simulink model "MPC"  (R2018a)
settings: Solver=VariableStepAuto  StartTime=0.0  StopTime=30  RelTol=1e-3
values from neighbouring files (symbols this model uses):
  I = 2500    [params.m]
  Kf = 55000    [params.m]
  Kr = 60000    [params.m]
  lf = 1.1    [params.m]
  lr = 1.6    [params.m]
  m = 1500    [params.m]
  n = 18.7    [params.m]
libraries: mpclib x1
settings Model: Creator=aoki-soya  LastModifiedBy=aoki-soya

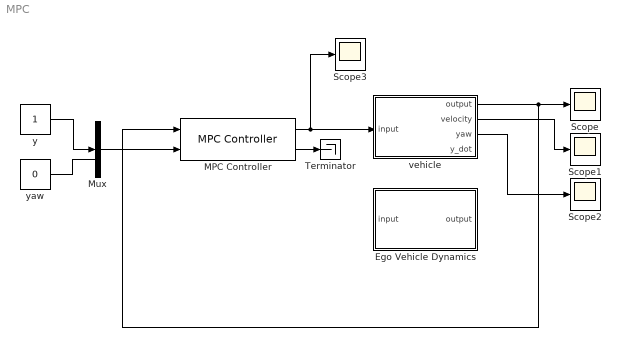
== system MPC ==
  Ego Vehicle Dynamics : Subsystem
  MPC Controller : mpclib/MPC Controller  SCDEnableBlockLinearizationSpecification=on  mpcobj=mpc1  is_multiple=0  enable_value=0  return_u0=off  updateMPCinCallerWorkspace=on  ref_from_ws=off  ref_signal_name=[]  ref_preview=off  md_from_ws=off  md_signal_name=[]  md_preview=off  from_project=off  project_file=MPCtask.mat  md_inport=off  mv_inport=off  cost_outport=on  return_sequence=off  return_qpstatus=off  return_state=off  state_inport=off  lims_inport=off  cc_inport=off  ywt_inport=off  is_designfromscratch=0  uwt_inport=off  duwt_inport=off  rhoeps_inport=off  uref_inport=off  n_ts=0.1  n_p=10  n_mv=2  n_md=0  n_ud=0  n_mo=1  n_uo=0  BlockDataType=double  SampleTimeInherited=off  switch_inport=off
  Mux : Mux  Inputs=1
  Scope{,1..3} (4 alike) : Scope
  Terminator : Terminator
  vehicle : Subsystem
  y : Constant
  yaw : Constant  Value=0
  wires:
  MPC Controller/1 -> Scope3/1, vehicle/1(input)
  vehicle/1(output) -> MPC Controller/1, Scope/1
  Mux/1 -> MPC Controller/2
  y/1 -> Mux/1
  yaw/1 -> ?
  MPC Controller/2 -> Terminator/1
  vehicle/2(velocity) -> Scope1/1
  vehicle/3(yaw) -> Scope2/1

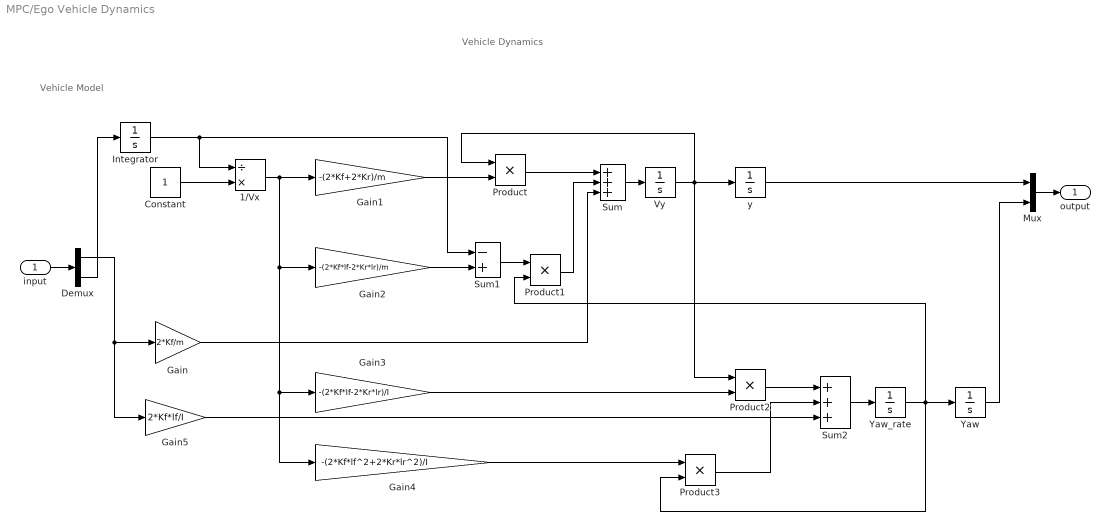
== system MPC/Ego Vehicle Dynamics ==
  note: Vehicle Model
  note: Vehicle Dynamics
  input : Inport
  1/Vx : Product  Inputs=/*
  Constant : Constant
  Demux : Demux  Outputs=2
  Gain : Gain  Gain=2*Kf/m
  Gain1 : Gain  Gain=-(2*Kf+2*Kr)/m
  Gain2 : Gain  Gain=-(2*Kf*lf-2*Kr*lr)/m
  Gain3 : Gain  Gain=-(2*Kf*lf-2*Kr*lr)/I
  Gain4 : Gain  Gain=-(2*Kf*lf^2+2*Kr*lr^2)/I
  Gain5 : Gain  Gain=2*Kf*lf/I
  Integrator : Integrator  InitialCondition=0.1  LimitOutput=on  LowerSaturationLimit=0.01
  Mux : Mux  Inputs=2
  Product{,1..3} (4 alike) : Product
  Sum : Sum  Inputs=+++
  Sum1 : Sum  Inputs=-+
  Sum2 : Sum  Inputs=+++
  Vy : Integrator
  Yaw : Integrator
  "Yaw_rate " : Integrator
  y : Integrator
  output : Outport
  wires:
  Sum2/1 -> "Yaw_rate "/1
  Gain2/1 -> Sum1/2
  Gain4/1 -> Product3/1
  Constant/1 -> 1/Vx/2
  Gain3/1 -> Product2/2
  1/Vx/1 -> Gain4/1, Gain3/1, Gain2/1, Gain1/1
  Product2/1 -> Sum2/1
  Product3/1 -> Sum2/2
  Gain5/1 -> Sum2/3
  Sum1/1 -> Product1/1
  "Yaw_rate "/1 -> Product3/2, Yaw/1, Product1/2
  Gain/1 -> Sum/3
  Demux/1 -> Gain/1, Gain5/1
  Gain1/1 -> Product/2
  Product/1 -> Sum/1
  Vy/1 -> Product/1, y/1, Product2/1
  Sum/1 -> Vy/1
  Demux/2 -> Integrator/1
  Product1/1 -> Sum/2
  Integrator/1 -> 1/Vx/1, Sum1/1
  Yaw/1 -> Mux/2
  Mux/1 -> output/1
  y/1 -> Mux/1
  input/1 -> Demux/1

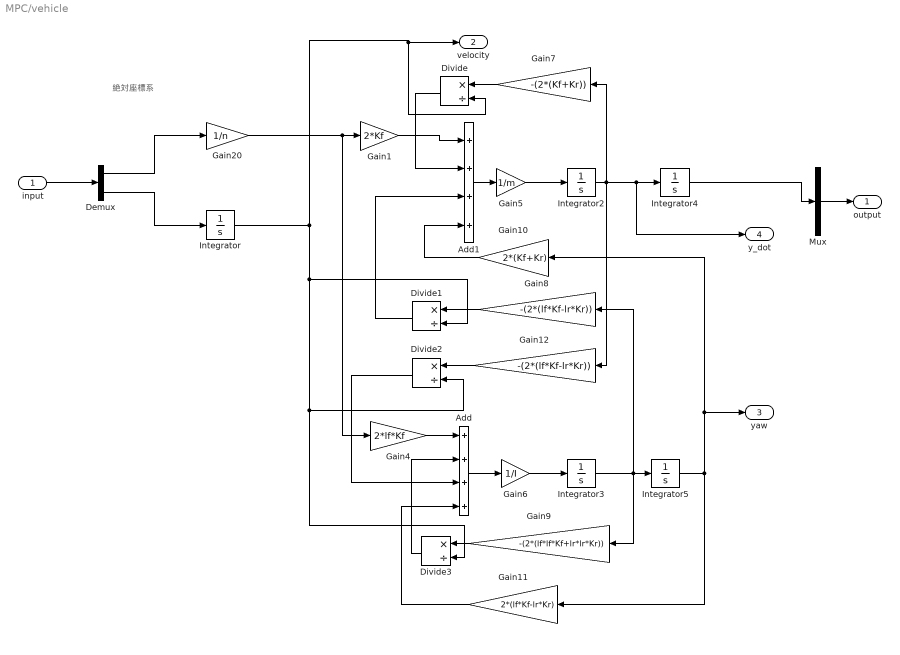
== system MPC/vehicle ==
  note: 絶対座標系
  input : Inport
  Add : Sum  Inputs=++++
  Add1 : Sum  Inputs=++++
  Demux : Demux  Outputs=2
  Divide{,1..3} (4 alike) : Product  Inputs=*/
  Gain1 : Gain  Gain=2*Kf
  Gain10 : Gain  Gain=2*(Kf+Kr)
  Gain11 : Gain  Gain=2*(lf*Kf-lr*Kr)
  Gain12 : Gain  Gain=-(2*(lf*Kf-lr*Kr))
  Gain20 : Gain  Gain=1/n
  Gain4 : Gain  Gain=2*lf*Kf
  Gain5 : Gain  Gain=1/m
  Gain6 : Gain  Gain=1/I
  Gain7 : Gain  Gain=-(2*(Kf+Kr))
  Gain8 : Gain  Gain=-(2*(lf*Kf-lr*Kr))
  Gain9 : Gain  Gain=-(2*(lf*lf*Kf+lr*lr*Kr))
  Integrator : Integrator  InitialCondition=0.1  LimitOutput=on  LowerSaturationLimit=0.0001
  Integrator{2..5} (4 alike) : Integrator
  Mux : Mux  Inputs=1
  output : Outport
  velocity : Outport  Port=2
  yaw : Outport  Port=3
  y_dot : Outport  Port=4
  wires:
  Gain6/1 -> Integrator3/1
  Integrator4/1 -> Mux/1
  Add/1 -> Gain6/1
  Gain10/1 -> Add1/4
  Add1/1 -> Gain5/1
  Gain11/1 -> Add/4
  Gain5/1 -> Integrator2/1
  Gain1/1 -> Add1/1
  Integrator3/1 -> Gain8/1, Integrator5/1, Gain9/1
  Integrator2/1 -> Gain7/1, Gain12/1, y_dot/1, Integrator4/1
  Gain4/1 -> Add/1
  Integrator5/1 -> Gain11/1, yaw/1, Gain10/1
  Demux/1 -> Gain20/1
  Gain20/1 -> Gain4/1, Gain1/1
  Demux/2 -> Integrator/1
  Mux/1 -> output/1
  input/1 -> Demux/1
  Divide/1 -> Add1/2
  Gain7/1 -> Divide/1
  Gain8/1 -> Divide1/1
  Divide1/1 -> Add1/3
  Gain12/1 -> Divide2/1
  Divide2/1 -> Add/3
  Gain9/1 -> Divide3/1
  Divide3/1 -> Add/2
  Integrator/1 -> Divide3/2, Divide2/2, Divide1/2, velocity/1, Divide/2
